simulink model "TVCRocketSimulation_Rev_1"  (R2021b)
settings: Solver=FixedStepAuto  StartTime=0.0  StopTime=2.4  FixedStep=1e-5  RelTol=1e-3
libraries: simulink_extras x3, slpidlib x1, shared3dof x1
settings Model: Creator=ian  LastModifiedBy=capn

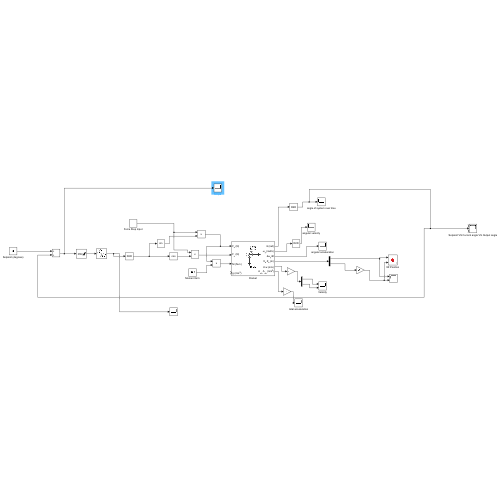
[thumbnail: Simulink's stored preview of the top-level diagram]
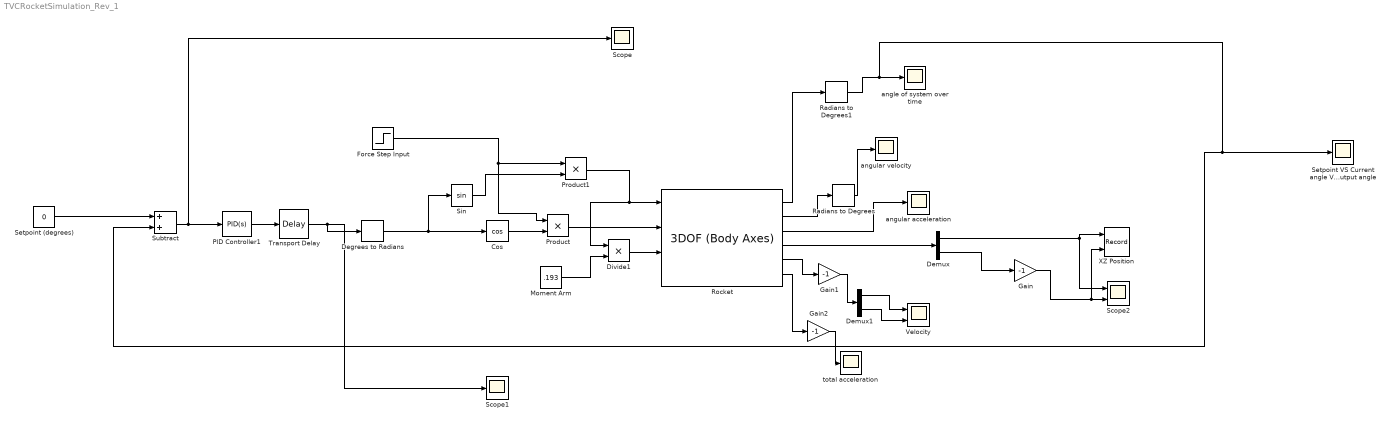
== system TVCRocketSimulation_Rev_1 ==
  Cos : Trigonometry  Operator=cos
  Degrees to Radians : simulink_extras/Transformations/Degrees to Radians
  Demux : Demux  Outputs=2
  Demux1 : Demux  Outputs=2
  Divide1 : Product  Inputs=**
  Force Step Input : Step  Time=2.4  Before=-15  After=0
  Gain : Gain  Gain=-1
  Gain1 : Gain  Gain=-1
  Gain2 : Gain  Gain=-1
  Moment Arm : Constant  Value=.193
  PID Controller1 : slpidlib/PID Controller  Controller=PID  Form=Parallel  TimeDomain=Continuous-time  UseExternalTs=off  SampleTime=-1  IntegratorMethod=Forward Euler  FilterMethod=Forward Euler  ControllerParametersSource=internal  P=3  I=0  D=1  UseFilter=on  N=100  TunerSelectOption=Transfer Function Based (PID Tuner App)  InitialConditionSource=internal  InitialConditionForIntegrator=0  InitialConditionForFilter=0  DifferentiatorICPrevScaledInput=0  ExternalReset=none  TrackingMode=off  Kt=1  LimitOutput=on  SatLimitsSource=internal  UpperSaturationLimit=5  LowerSaturationLimit=-5  LinearizeAsGain=on  AntiWindupMode=none  Kb=1  POutMin=[]  POutMax=[]  IOutMin=[]  IOutMax=[]  DOutMin=[]  DOutMax=[]  NOutMin=[]  NOutMax=[]  SumOutMin=[]  SumOutMax=[]  SaturationOutMin=[]  SaturationOutMax=[]  PParamMin=[]  PParamMax=[]  IParamMin=[]  IParamMax=[]  DParamMin=[]  DParamMax=[]  NParamMin=[]  NParamMax=[]  KbParamMin=[]  KbParamMax=[]  KtParamMin=[]  KtParamMax=[]  KbOutMin=[]  KbOutMax=[]  KtOutMin=[]  KtOutMax=[]  IntegratorOutMin=[]  IntegratorOutMax=[]  FilterOutMin=[]  FilterOutMax=[]  SumI1OutMin=[]  SumI1OutMax=[]  SumI2OutMin=[]  SumI2OutMax=[]  SumI3OutMin=[]  SumI3OutMax=[]  SumI4OutMin=[]  SumI4OutMax=[]  SumDOutMin=[]  SumDOutMax=[]  DifferentiatorOutMin=[]  DifferentiatorOutMax=[]  FilterDiffOutCoefMin=[]  FilterDiffOutCoefMax=[]  ReciprocalOutMin=[]  ReciprocalOutMax=[]  SumDenOutMin=[]  SumDenOutMax=[]  SumNumOutMin=[]  SumNumOutMax=[]  DivideOutMin=[]  DivideOutMax=[]  UdiffTsProdOutMin=[]  UdiffTsProdOutMax=[]  NTsProdOutMin=[]  NTsProdOutMax=[]  UintegralTsProdOutMin=[]  UintegralTsProdOutMax=[]  UngainTsProdOutMin=[]  UngainTsProdOutMax=[]  IntegratorContinuousStateAttributes=''  IntegratorStateMustResolveToSignalObject=off  IntegratorRTWStateStorageClass=Auto  FilterContinuousStateAttributes=''  FilterStateMustResolveToSignalObject=off  FilterRTWStateStorageClass=Auto  ParallelPVariant=InternalParameters  IdealPVariant=Disabled  IVariant=InternalParameters  DVariant=InternalParameters  IntegratorVariant=Continuous  SatVariant=Enabled  AWVariant=Passthrough  PCopyVariant=Disabled  TRVariant=Disabled  FdbkBlocksVariant=Forward  IdealPFdbkVariant=Disabled  SatFdbkVariant=Disabled  DerivativeFilterVariant=ContFilter  NVariant=InternalParameters  NCopyVariant=Disabled  FilterICVariant=InternalICsFilter  IntegratorICVariant=InternalICs  ExternalResetVariant=Disabled  TRSumVariant=Passthrough  SumFdbkVariant=Disabled  SumVariant=Sum_PID  TsampFilterVariant=InternalTs  TsampNgainVariant=Passthrough  TsampIntegralVariant=Passthrough  ExternalSaturationOutDataTypeStr=Inherit: Same as second input
  Product : Product  RndMeth=Zero
  Product1 : Product  RndMeth=Zero
  Radians to Degrees : simulink_extras/Transformations/Radians to Degrees
  Radians to Degrees1 : simulink_extras/Transformations/Radians to Degrees
  Rocket : shared3dof/3DOF (Body Axes)  units=Metric (MKS)  mtype=Fixed  v_ini=0  theta_ini=pi/100  alpha_ini=0  pos_ini=[0 0]  q_ini=0  mass=.805  mass_e=0.5  mass_f=3.0  Iyy=.017  Iyy_e=0.5  Iyy_f=3.0  g_in=External  g=9.81  vre_flag=on  abi_flag=off  aMode=0  vel_statename=''  theta_statename=''  pos_statename=''  q_statename=''  mass_statename=''
      settings: SourceProductBaseCode=AE,PW,DR,MT,UV,VE
  Scope : Scope
  Scope1 : Scope
  Scope2 : Scope  NumInputPorts=2
  Setpoint (degrees) : Constant  Value=0
  Setpoint VS Current angle VS Output angle : Scope  NumInputPorts=3
  Sin : Trigonometry
  Subtract : Sum
  Transport Delay : TransportDelay  DelayTime=0.005
  Velocity : Scope  NumInputPorts=2
  XZ Position : Record  FileSettingsInternal="{\"entries\":[{\"content\":{\"excelSettings\":{\"content\":{},\"type\":\"Streamout.ExcelSettings\"}},\"type\":\"Streamout.FileSettingStorage\",\"uuid\":\"223a5e4b-58bf-420d-9902-a4892c3d334a\"}],\"packageUris\":[\"http://schema.mathworks.com/mf0/streamout_blocks/R2020a\"],\"version\":\"1.0\"}"  Layout=[1 1]  SignalsInternal="{\"entries\":[{\"content\":{\"signals\":[{\"content\":{\"blockPath\":[\"TVCRocketSimulation/XZ Position\"],\"channel\":[],\"dimensions\":[1],\"domain\":\"TVCRocketSimulation/XZ Position\",\"lineColor\":\"#a2142f\",\"plots\":[1],\"port\":1,\"sid\":[\"\"],\"signalID\":2037,\"signalName\":\"Demux:1\"},\"type\":\"RecordBlkView.Signal\",\"uuid\":\"9a38a8ca-a9e1-45f4-99b9-63b4e1d8122a\"},{\"content\":{\"blockPath\":[\"TVCRocketSimulation/XZ Position\"],\"channel\":[],\"dimensions\":[1],\"domain\":\"TVCRocketSimulation/XZ Position\",\"lineColor\":\"#139fff\",\"plots\":[1],\"port\":2,\"sid\":[\"\"],\"signalID\":2041,\"signalName\":\"Gain\"},\"type\":\"RecordBlkView.Signal\",\"uuid\":\"21b67e6c-72c2-4358-a77d-b3be59f68f38\"}]},\"type\":\"RecordBlkView.InputSignals\",\"uuid\":\"a7c36b2e-2c8f-42d7-b435-97eba4b05579\"}],\"packageUris\":[\"http://schema.mathworks.com/mf0/streamout_blocks/R2020a\"],\"version\":\"1.0\"}"  VisualizationBindings="{\"xyplotplugin\":{\"info\":[{\"series\":[{\"bindingParametersList\":[{\"parameter\":\"X-Axis\",\"signalID\":2037,\"signalName\":\"Demux:1\"},{\"parameter\":\"Y-Axis\",\"signalID\":2041,\"signalName\":\"Gain\"}],\"seriesID\":1101}],\"subplotID\":1}]}}"  CompatibilityTag=XY  st=-1
  angle of system over time : Scope
  angular acceleration : Scope
  angular velocity : Scope
  total acceleration : Scope
  wires:
  Rocket/4 -> Demux/1
  Demux/1 -> Scope2/1, XZ Position/1
  Force Step Input/1 -> Product1/1, Product/1
  Cos/1 -> Product/2
  Product1/1 -> Rocket/1, Divide1/1
  Sin/1 -> Product1/2
  Product/1 -> Rocket/2
  Moment Arm/1 -> Divide1/2
  Degrees to Radians/1 -> Cos/1, Sin/1
  Demux/2 -> Gain/1
  Gain/1 -> Scope2/2, XZ Position/2
  Divide1/1 -> Rocket/3
  Rocket/1 -> Radians to Degrees1/1
  Rocket/6 -> Gain2/1
  Rocket/5 -> Gain1/1
  Demux1/1 -> Velocity/1
  Demux1/2 -> Velocity/2
  Gain1/1 -> Demux1/1
  Gain2/1 -> total acceleration/1
  Rocket/3 -> angular acceleration/1
  Rocket/2 -> Radians to Degrees/1
  Radians to Degrees/1 -> angular velocity/1
  PID Controller1/1 -> Transport Delay/1
  Subtract/1 -> Scope/1, PID Controller1/1
  Radians to Degrees1/1 -> Setpoint VS Current angle VS Output angle/2, Subtract/2, angle of system over time/1
  Setpoint (degrees)/1 -> Subtract/1
  Transport Delay/1 -> Scope1/1, Degrees to Radians/1
